simulink model "PF_FeedForward_Control"  (R2015a)
settings: Solver=ode45  StartTime=0.0  StopTime=10.0  RelTol=1e-3
values from neighbouring files (symbols this model uses):
  ddq = diff([zeros(1,n); dq])./diff(tm)    [PF_Parametrised_clv_Traj.m]    (also in PF_Table_clv_Traj.m; PF_Uncoodinated_Traj.m = zeros(sp,n))
  dq = y(:,n+1:2*n)    [PF_Forward_Dynamics.m]    (also in PF_Inverse_Kinematics.m = Jinv * r'; PF_Parametrised_clv_Traj.m = diff([zeros(1,n); q])./diff(tm); PF_Table_clv_Traj.m = diff([zeros(1,n); q])./diff(tm); PF_Uncoodinated_Traj.m = zeros(sp,n))
  q = S.value{'home_q'}    [MF_Save_Settings.m]    (also in PF_Forward_Dynamics.m = q(:)'; PF_Forward_Kinematics.m = deg2rad(q); PF_Inverse_Kinematics.m = q + dq'; PF_Parametrised_clv_Traj.m = PF_Inverse_Kinematics(p, q0, s))
  q0 = [q0(:); qd0(:)]    [PF_Forward_Dynamics.m]    (also in PF_Inverse_Kinematics.m = q; PF_Parametrised_clv_Traj.m = H(cn - 1).q(end,:); PF_Table_clv_Traj.m = H(cn - 1).q(end,:); PF_Uncoodinated_Traj.m = H(cn - 1).q(end,:))
undefined symbols (not defined in the file or in its folder): PF_Inverse_DynamicsII
settings Model: Creator=Diego  LastModifiedBy=Diego

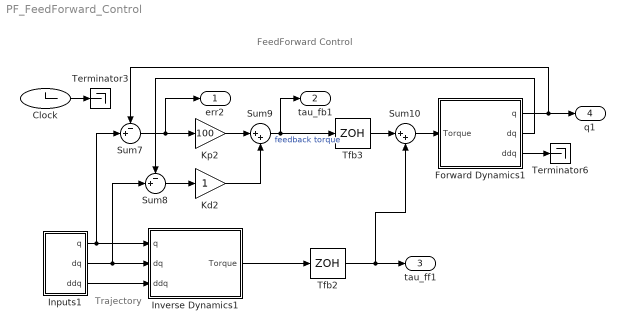
== system PF_FeedForward_Control ==
  note: Trajectory
  note: FeedForward Control
  Clock : Clock
  Forward Dynamics1 : Subsystem
  Inputs1 : Subsystem
  Inverse Dynamics1 : Subsystem
  Kd2 : Gain  SaturateOnIntegerOverflow=on  OutDataTypeStr=Inherit: Same as input  ParamDataTypeStr=Inherit: Same as input
  Kp2 : Gain  Gain=100  SaturateOnIntegerOverflow=on  OutDataTypeStr=Inherit: Same as input  ParamDataTypeStr=Inherit: Same as input
  Sum10 : Sum  Inputs=|++  SaturateOnIntegerOverflow=on  InputSameDT=on  OutDataTypeStr=Inherit: Same as first input
  Sum7 : Sum  Inputs=-+|  SaturateOnIntegerOverflow=on  InputSameDT=on  OutDataTypeStr=Inherit: Same as first input
  Sum8 : Sum  Inputs=-+|  SaturateOnIntegerOverflow=on  InputSameDT=on  OutDataTypeStr=Inherit: Same as first input
  Sum9 : Sum  Inputs=|++  SaturateOnIntegerOverflow=on  InputSameDT=on  OutDataTypeStr=Inherit: Same as first input
  Terminator3 : Terminator
  Terminator6 : Terminator
  Tfb2 : ZeroOrderHold  SampleTime=0.01
  Tfb3 : ZeroOrderHold  SampleTime=0.01
  err2 : Outport
  tau_fb1 : Outport  Port=2
  tau_ff1 : Outport  Port=3
  q1 : Outport  Port=4
  wires:
  Inverse Dynamics1/1(Torque) -> Tfb2/1
  Inputs1/3(ddq) -> Inverse Dynamics1/3(ddq)
  Kd2/1 -> Sum9/2
  Sum7/1 -> Kp2/1, err2/1
  Kp2/1 -> Sum9/1
  Sum8/1 -> Kd2/1
  Sum9/1 -> Tfb3/1, tau_fb1/1  "feedback torque"
  Sum10/1 -> Forward Dynamics1/1(Torque)
  Forward Dynamics1/1(q) -> q1/1, Sum7/1
  Forward Dynamics1/2(dq) -> Sum8/1
  Inputs1/1(q) -> Sum7/2, Inverse Dynamics1/1(q)
  Inputs1/2(dq) -> Sum8/2, Inverse Dynamics1/2(dq)
  Tfb2/1 -> Sum10/2, tau_ff1/1
  Tfb3/1 -> Sum10/1
  Forward Dynamics1/3(ddq) -> Terminator6/1
  Clock/1 -> Terminator3/1

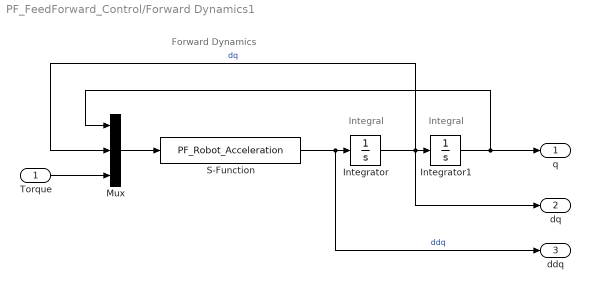
== system PF_FeedForward_Control/Forward Dynamics1 ==
  note: Forward Dynamics
  note: Integral
  note: Integral
  Torque : Inport
  Integrator : Integrator
  Integrator1 : Integrator  InitialCondition=q0
  Mux : Mux  Inputs=3
  S-Function : S-Function  FunctionName=PF_Robot_Acceleration  Parameters=robot
  q : Outport
  dq : Outport  Port=2
  ddq : Outport  Port=3
  wires:
  Torque/1 -> Mux/3
  Mux/1 -> S-Function/1
  S-Function/1 -> ddq/1, Integrator/1  "ddq"
  Integrator/1 -> dq/1, Integrator1/1, Mux/2  "dq"
  Integrator1/1 -> q/1, Mux/1

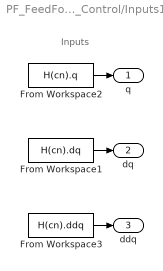
== system PF_FeedForward_Control/Inputs1 ==
  note: Inputs
  From Workspace1 : FromWorkspace  VariableName=H(cn).dq  SampleTime=0.1
  From Workspace2 : FromWorkspace  VariableName=H(cn).q  SampleTime=0.1
  From Workspace3 : FromWorkspace  VariableName=H(cn).ddq  SampleTime=0.1
  q : Outport
  dq : Outport  Port=2
  ddq : Outport  Port=3
  wires:
  From Workspace1/1 -> dq/1
  From Workspace3/1 -> ddq/1
  From Workspace2/1 -> q/1

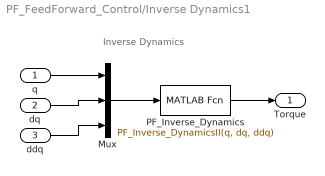
== system PF_FeedForward_Control/Inverse Dynamics1 ==
  note: Inverse Dynamics
  q : Inport
  dq : Inport  Port=2
  ddq : Inport  Port=3
  Mux : Mux  Inputs=3
  PF_Inverse_Dynamics : MATLABFcn  MATLABFcn=PF_Inverse_DynamicsII(q, dq, ddq)  OutputDimensions=n
  Torque : Outport
  wires:
  PF_Inverse_Dynamics/1 -> Torque/1
  Mux/1 -> PF_Inverse_Dynamics/1
  q/1 -> Mux/1
  dq/1 -> Mux/2
  ddq/1 -> Mux/3
